simulink model "pdl_nonlinear_hw3n"  (R2017a)
settings: Solver=VariableStepAuto  StartTime=0.0  StopTime=duration  RelTol=1e-3
values from neighbouring files (symbols this model uses):
  b = 0.1    [pendulum_hw3linear.m]    (also in pendulum_hw3nonlinear.m)
  C = [1 0 0 0; 0 1 0 0]    [pendulum_hw3linear.m]    (also in pendulum_hw3nonlinear.m)
  f_p = 1e-4    (= 0.0001)    [pendulum_hw3linear.m]    (also in pendulum_hw3nonlinear.m)
  g = 9.81    [pendulum_hw3linear.m]    (also in pendulum_hw3nonlinear.m)
  K = lqr(A_a,B_a,Q,R)    [pendulum_hw3linear.m]    (also in pendulum_hw3nonlinear.m = lqr(A,B,Q,R))
  k = 0.15    [pendulum_hw3linear.m]    (also in pendulum_hw3nonlinear.m)
  L = 1.4    [pendulum_hw3linear.m]    (also in pendulum_hw3nonlinear.m)
  m = 0.75    [pendulum_hw3linear.m]    (also in pendulum_hw3nonlinear.m)
  M = 1    [pendulum_hw3linear.m]    (also in pendulum_hw3nonlinear.m)
  m_p = 1e-7    (= 1e-07)    [pendulum_hw3linear.m]    (also in pendulum_hw3nonlinear.m)
  Nbar = -pinv(B_a)*A_a*pinv(Cn)+K*pinv(Cn)    [pendulum_hw3linear.m]    (also in pendulum_hw3nonlinear.m = -pinv(B)*A*pinv(Cn)+K*pinv(Cn))
  Q_k = diag([1 1])    [pendulum_hw3linear.m]    (also in pendulum_hw3nonlinear.m)
  R_k = 1e-4*diag([1 1])    [pendulum_hw3linear.m]    (also in pendulum_hw3nonlinear.m)
  Ts = 0.001    [pendulum_hw3linear.m]    (also in pendulum_hw3nonlinear.m)
  w_p = 10    [pendulum_hw3linear.m]    (also in pendulum_hw3nonlinear.m)
undefined symbols (not defined in the file or in its folder): Delta, Gamma, Phi
libraries: simulink x3, simulink_extras x2
settings Model: Creator=Salmon  LastModifiedBy=Salmon

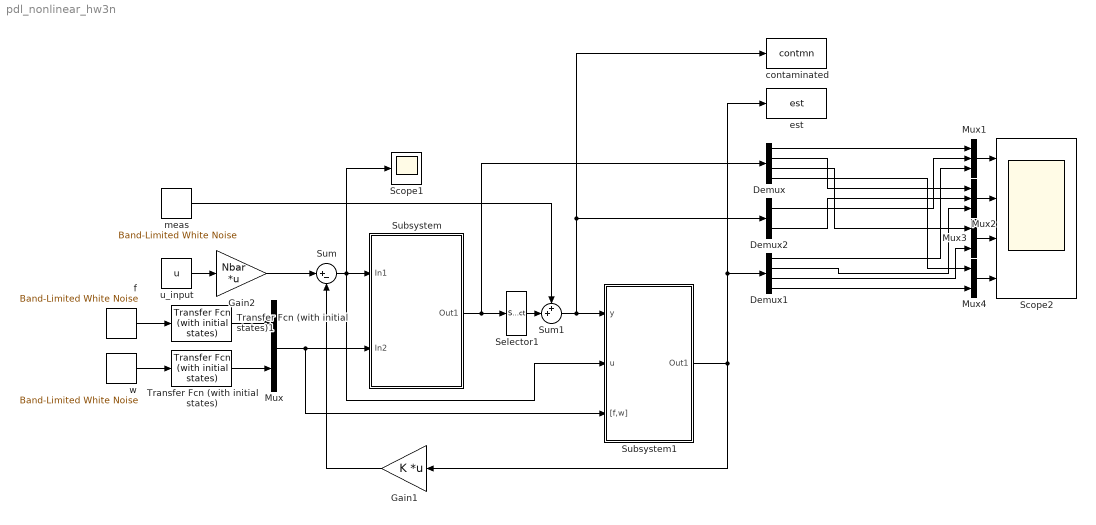
== system pdl_nonlinear_hw3n ==
  Demux : Demux
  Demux1 : Demux
  Demux2 : Demux  Outputs=2
  Gain1 : Gain  Gain=K  Multiplication=Matrix(K*u)
  Gain2 : Gain  Gain=Nbar  Multiplication=Matrix(K*u)
  Mux : Mux  Inputs=2
  Mux1 : Mux  Inputs=3
  Mux2 : Mux  Inputs=3
  Mux3 : Mux  Inputs=2
  Mux4 : Mux  Inputs=2
  Scope1 : Scope
  Scope2 : Scope  NumInputPorts=4
  Selector1 : Selector  InputPortWidth=4  IndexOptions=Index vector (dialog)  Indices=[1 2]  OutputSizes=1
  Subsystem : Subsystem
  Subsystem1 : Subsystem
  Sum : Sum  Inputs=|+-
  Sum1 : Sum  Inputs=++|
  Transfer Fcn (with initial states) : simulink_extras/Additional Linear/Transfer Fcn (with initial states)  N=[0.64]  D="[1  0.8]"  X0=0
  Transfer Fcn (with initial states)1 : simulink_extras/Additional Linear/Transfer Fcn (with initial states)  N=[0.64]  D="[1  0.8]"  X0=0
  contaminated : ToWorkspace  VariableName=contmn  SaveFormat=Structure With Time  SampleTime=Ts
  est : ToWorkspace  VariableName=est  SaveFormat=Structure With Time  SampleTime=Ts
  f : simulink/Sources/Band-Limited White Noise  Cov=[f_p]  Ts=Ts  seed=[23341]
  meas : simulink/Sources/Band-Limited White Noise  Cov=[m_p,m_p]  Ts=Ts  seed=[123,23341]
  u_input : Constant  Value=u
  w : simulink/Sources/Band-Limited White Noise  Cov=[w_p]  Ts=Ts  seed=[23341]
  wires:
  u_input/1 -> Gain2/1
  f/1 -> Transfer Fcn (with initial states)1/1
  w/1 -> Transfer Fcn (with initial states)/1
  Mux/1 -> Subsystem1/3("[f,w]"), Subsystem/2(In2)
  Gain1/1 -> Sum/2
  Gain2/1 -> Sum/1
  Demux/3 -> Mux3/1
  Mux1/1 -> Scope2/1
  Demux/4 -> Mux4/1
  Demux2/2 -> Mux2/2
  Mux4/1 -> Scope2/4
  Demux1/1 -> Mux1/3
  Demux/1 -> Mux1/1
  Subsystem/1(Out1) -> Demux/1, Selector1/1
  Mux2/1 -> Scope2/2
  Demux1/4 -> Mux4/2
  Sum1/1 -> contaminated/1, Demux2/1, Subsystem1/1(y)
  Selector1/1 -> Sum1/2
  meas/1 -> Sum1/1
  Demux/2 -> Mux2/1
  Demux1/2 -> Mux2/3
  Sum/1 -> Subsystem1/2(u), Scope1/1, Subsystem/1(In1)
  Demux1/3 -> Mux3/2
  Mux3/1 -> Scope2/3
  Demux2/1 -> Mux1/2
  Subsystem1/1(Out1) -> est/1, Demux1/1, Gain1/1
  Transfer Fcn (with initial states)/1 -> Mux/2
  Transfer Fcn (with initial states)1/1 -> Mux/1

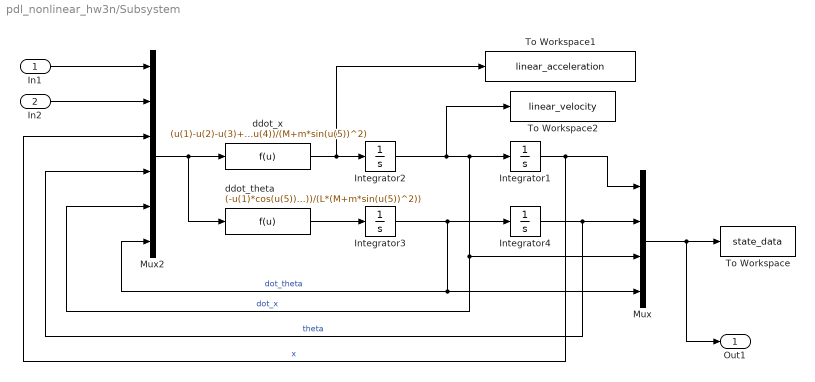
== system pdl_nonlinear_hw3n/Subsystem ==
  In1 : Inport
  In2 : Inport  Port=2
  Integrator{1..4} (4 alike) : Integrator
  Mux : Mux
  Mux2 : Mux  Inputs=6
  To Workspace : ToWorkspace  VariableName=state_data  SaveFormat=Structure With Time  SampleTime=-1
  To Workspace1 : ToWorkspace  VariableName=linear_acceleration  SaveFormat=Structure With Time  SampleTime=-1
  To Workspace2 : ToWorkspace  VariableName=linear_velocity  SaveFormat=Structure With Time  SampleTime=-1
  ddot_theta : Fcn  Expr=(-u(1)*cos(u(5))+u(3)*cos(u(5))-m*L*u(7)^2*sin(u(5))*cos(u(5))+(M+m)*g*sin(u(5))-(M/m)*u(2)*cos(u(5))+b*u(6)*cos(u(5))+k*u(4)*cos(u(5)))/(L*(M+m*sin(u(5))^2))
  ddot_x : Fcn  Expr=(u(1)-u(2)-u(3)+u(2)*cos(u(5))^2+m*L*u(7)^2*sin(u(5))-m*g*sin(u(5))*cos(u(5))-b*u(6)-k*u(4))/(M+m*sin(u(5))^2)
  Out1 : Outport
  wires:
  Integrator3/1 -> Mux2/6, Mux/4, Integrator4/1  "dot_theta"
  In2/1 -> Mux2/2
  ddot_x/1 -> To Workspace1/1, Integrator2/1
  Integrator2/1 -> To Workspace2/1, Mux2/5, Mux/3, Integrator1/1  "dot_x"
  ddot_theta/1 -> Integrator3/1
  Mux/1 -> Out1/1, To Workspace/1
  In1/1 -> Mux2/1
  Integrator1/1 -> Mux2/3, Mux/1  "x"
  Mux2/1 -> ddot_theta/1, ddot_x/1
  Integrator4/1 -> Mux2/4, Mux/2  "theta"

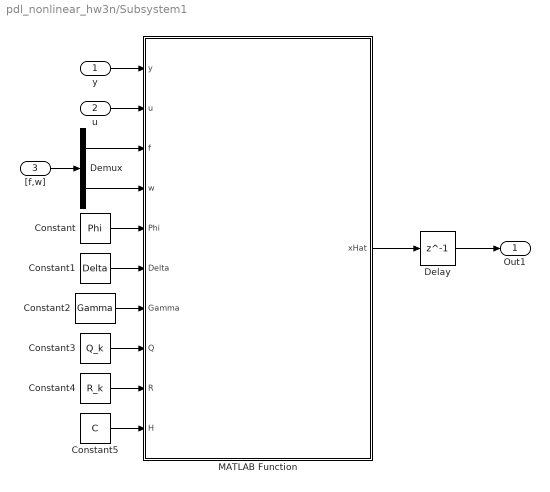
== system pdl_nonlinear_hw3n/Subsystem1 ==
  y : Inport
  u : Inport  Port=2
  "[f,w]" : Inport  Port=3
  Constant : Constant  Value=Phi
  Constant1 : Constant  Value=Delta
  Constant2 : Constant  Value=Gamma
  Constant3 : Constant  Value=Q_k
  Constant4 : Constant  Value=R_k
  Constant5 : Constant  Value=C
  Delay : Delay  DelayLength=1  InitialCondition=0
  Demux : Demux  Outputs=2
  MATLAB Function : MATLAB Function  TreatAsAtomicUnit=on
  Out1 : Outport
  wires:
  y/1 -> MATLAB Function/1(y)
  MATLAB Function/1(xHat) -> Delay/1
  u/1 -> MATLAB Function/2(u)
  Constant/1 -> MATLAB Function/5(Phi)
  Constant1/1 -> MATLAB Function/6(Delta)
  Constant3/1 -> MATLAB Function/8(Q)
  Constant2/1 -> MATLAB Function/7(Gamma)
  Constant4/1 -> MATLAB Function/9(R)
  Constant5/1 -> MATLAB Function/10(H)
  Delay/1 -> Out1/1
  Demux/1 -> MATLAB Function/3(f)
  Demux/2 -> MATLAB Function/4(w)
  "[f,w]"/1 -> Demux/1

== matlab function pdl_nonlinear_hw3n/Subsystem1/MATLAB Function ==
  data: y input; u input; f input; w input; xHat output; Phi input; Delta input; Gamma input; Q input; R input; H input
function xHat = fcn(y,u,f,w,Phi,Delta,Gamma,Q,R,H)

M = 1;                  %[kg]    cart mass
m = 0.75;               %[kg]    pendulum mass
b = 0.1;                %[N·s/m] damper coefficient
k = 0.15;               %[N/m]   spring stiffness
sat_linear = 5*pi/180;  %[rad]   linear saturation for theta in linear model
sat_nl = pi/2;          %[raf]   saturation for theta in nonlinear model
g = 9.81;               %[m/s^2] gravitational acceleration
L = 1.4;                %[m]     Presumed rod length for linearized model
Ts = 0.001;              %[s]     sampling time

persistent Pbar xbar

% init. Pbar xbar
if isempty(Pbar)
    Pbar = 1e-6*eye(4);
end

if isempty(xbar)
    xbar = zeros(4,1);
end

% 1. Kalman gain
K = Pbar*H'*[H*Pbar*H'+R]^(-1);

% 2. state est. update
xHat = xbar + K*[y-H*xbar];

% 3. error covariance update
Phat = [eye(4)-K*H]*Pbar*[eye(4)-K*H]'+K*R*K';

% 4. state est. propagation
%xbar = Phi*xHat+Delta*u;
xbar = xHat + Ts*[xHat(3); xHat(4);(u-f-w+f*cos(xHat(2))^2+m*L*xHat(4)^2*sin(xHat(2))-m*g*sin(xHat(2))*cos(xHat(2))-b*xHat(3)-k*xHat(1))/(M+m*sin(xHat(2))^2);(-u*cos(xHat(2))+w*cos(xHat(2))-m*L*xHat(4)^2*sin(xHat(2))*cos(xHat(2))+(m+M)*g*sin(xHat(2))-M*f*cos(xHat(2))/m+b*xHat(3)*cos(xHat(2))+k*xHat(1)*cos(xHat(2)))/(L*(M+m*sin(xHat(2))^2))];

% 5. error covariance propagation
Pbar = Phi*Phat*Phi'+Gamma*Q*Gamma';
